simulink model "k1"  (Simulink 7.3)
settings: Solver=ode23t  StartTime=0.0  StopTime=10.0  RelTol=1e-9
libraries: simulink x2
settings Model: Creator=Sainquake  LastModifiedBy=Sainquake

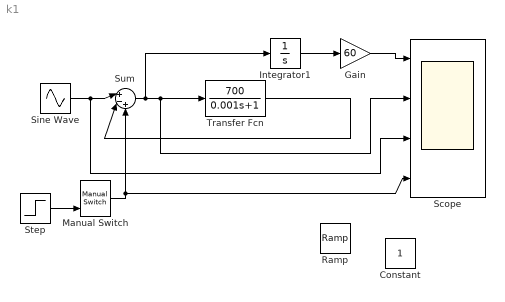
== system k1 ==
  Constant : Constant  OutDataType=fixdt(1, 16)  OutScaling=2^0
  Gain : Gain  Gain=60  ParameterDataType=fixdt(1, 16)  ParameterScaling=2^0  OutDataType=fixdt(1, 16)  OutScaling=2^0
  Integrator1 : Integrator
  Manual Switch : simulink/Signal Routing/Manual Switch  SystemSampleTime=-1  sw=0  action=0  varsize=off
  Ramp : simulink/Sources/Ramp  SystemSampleTime=-1  slope=1  start=0  X0=0
  Scope : Scope  NumInputPorts=4
      settings: YMin=-5~-5~-5~-5  YMax=5~5~5~5  MaxDataPoints=500000000
  Sine Wave : Sin  Amplitude=31.5  Bias=0  Frequency=1.25  Phase=0  Samples=10  SampleTime=0  Offset=0
  Step : Step  After=5  SampleTime=0
  Sum : Sum  Inputs=|+-+  OutDataType=fixdt(1, 16)  OutScaling=2^0
  Transfer Fcn : TransferFcn  Numerator=[700]  Denominator=[0.001 1]
  wires:
  Transfer Fcn/1 -> Sum/2
  Sum/1 -> Transfer Fcn/1, Scope/2, Integrator1/1
  Sine Wave/1 -> Sum/1, Scope/3
  Gain/1 -> Scope/1
  Step/1 -> Manual Switch/2
  Manual Switch/1 -> Sum/3, Scope/4
  Integrator1/1 -> Gain/1
